simulink model "sunsensor_error_test"  (R2018b)
settings: Solver=VariableStepAuto  StartTime=0.0  StopTime=1000  RelTol=1e-3
undefined symbols (not defined in the file): simParams
libraries: simulink x2, dspswit3 x2, dspstat3 x2, MEKF_Conversion_lib x2
settings Model: Creator=Taylor  LastModifiedBy=Taylor

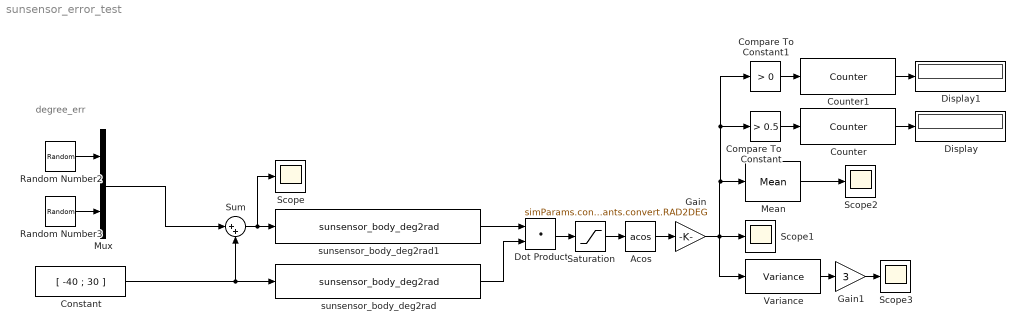
== system sunsensor_error_test ==
  note: degree_err
  Acos : Trigonometry  Operator=acos
  Compare To Constant : simulink/Logic and Bit Operations/Compare To Constant  relop=>  const=0.5  OutDataTypeStr=boolean
  Compare To Constant1 : simulink/Logic and Bit Operations/Compare To Constant  relop=>  const=0  OutDataTypeStr=boolean
  Constant : Constant  Value=[ -40 ; 30 ]
  Counter : dspswit3/Counter  Direction=Up  CountEvent=Rising edge  CounterSize=32 bits  MaxCount=255  InitialCount=0  Output=Count  HitValue=32  ResetInput=off  SamplesPerFrame=1  Ts=1  CntDtype=double  HitDtype=Logical
  Counter1 : dspswit3/Counter  Direction=Up  CountEvent=Non-zero sample  CounterSize=32 bits  MaxCount=255  InitialCount=0  Output=Count  HitValue=32  ResetInput=off  SamplesPerFrame=1  Ts=1  CntDtype=double  HitDtype=Logical
  Display : Display
  Display1 : Display
  Dot Product : DotProduct  InputSameDT=on  OutDataTypeStr=Inherit: Inherit via internal rule
  Gain : Gain  Gain=simParams.constants.convert.RAD2DEG
  Gain1 : Gain  Gain=3
  Mean : dspstat3/Mean  run=on  InputProcessing=Columns as channels (frame based)  reset_popup=None  directionMode=Each column  dimension=1  roiEnable=off  roiType=Rectangles  roiPortion=Entire ROI  roiOutput=Individual statistics for each ROI  roiFlag=off  roundingMode=Floor  overflowMode=off  outputDataTypeStr=Inherit: Same as accumulator  outputMin=[]  outputMax=[]  outputLastDataTypeStr=Inherit: Same as accumulator
  Mux : Mux  Inputs=2
  Random Number2 : RandomNumber  Variance=simParams.sensors.sun_sensor.deg_var  Seed=simParams.sensors.sun_sensor.seed(1)  SampleTime=simParams.sensors.sun_sensor.sample_time_s
  Random Number3 : RandomNumber  Variance=simParams.sensors.sun_sensor.deg_var  Seed=simParams.sensors.sun_sensor.seed(2)  SampleTime=simParams.sensors.sun_sensor.sample_time_s
  Saturation : Saturate  UpperLimit=1  LowerLimit=-1
  Scope{,1..3} (4 alike) : Scope
  Sum : Sum  Inputs=|++
  Variance : dspstat3/Variance  run=on  InputProcessing=Columns as channels (frame based)  reset_popup=None  directionMode=Each column  dimension=1  roiEnable=off  roiType=Rectangles  roiPortion=Entire ROI  roiOutput=Individual statistics for each ROI  roiFlag=off  roundingMode=Floor  overflowMode=off
      settings: SourceProductName=DSP System Toolbox
  sunsensor_body_deg2rad : MEKF_Conversion_lib/Conversion_lib/sunsensor_body_deg2rad  SystemSampleTime=-1
  sunsensor_body_deg2rad1 : MEKF_Conversion_lib/Conversion_lib/sunsensor_body_deg2rad  SystemSampleTime=-1
  wires:
  Mux/1 -> Sum/1
  Constant/1 -> sunsensor_body_deg2rad/1, Sum/2
  Sum/1 -> Scope/1, sunsensor_body_deg2rad1/1
  sunsensor_body_deg2rad1/1 -> Dot Product/1
  sunsensor_body_deg2rad/1 -> Dot Product/2
  Dot Product/1 -> Saturation/1
  Saturation/1 -> Acos/1
  Acos/1 -> Gain/1
  Gain/1 -> Compare To Constant1/1, Compare To Constant/1, Mean/1, Variance/1, Scope1/1
  Mean/1 -> Scope2/1
  Variance/1 -> Gain1/1
  Gain1/1 -> Scope3/1
  Compare To Constant/1 -> Counter/1
  Counter/1 -> Display/1
  Compare To Constant1/1 -> Counter1/1
  Counter1/1 -> Display1/1
  Random Number2/1 -> Mux/1
  Random Number3/1 -> Mux/2
